simulink model "sat"  (R2019b)
settings: Solver=VariableStepAuto  StartTime=0.0  StopTime=T  RelTol=1e-3
values from neighbouring files (symbols this model uses):
  a0 = 2*Q + sinw    [filter_plot.m]    (also in sat_sim.m = (1 - cosw + sinw))
  a1 = -4*Q*cosw    [filter_plot.m]    (also in sat_sim.m = 2 * ( 1 - cosw))
  a2 = 2*Q - sinw    [filter_plot.m]    (also in sat_sim.m = 1 - cosw - sinw)
  b0 = Q*sinw    [filter_plot.m]    (also in sat_sim.m = 1 - cosw)
  b1 = 0    [filter_plot.m]    (also in sat_sim.m = 2 * b0)
  b2 = -Q*sinw    [filter_plot.m]    (also in sat_sim.m = b0)
  fs = 44100    [filter_plot.m]    (also in plot_adsr.m; plot_spectrogram.m; plot_waveform.m; sat_sim.m)
  G = 10.0    (= 10)    [sat_sim.m]
libraries: dspsrcs4 x3
settings Model: SimulationMode=rapid-accelerator  Creator=27849  LastModifiedBy=27849

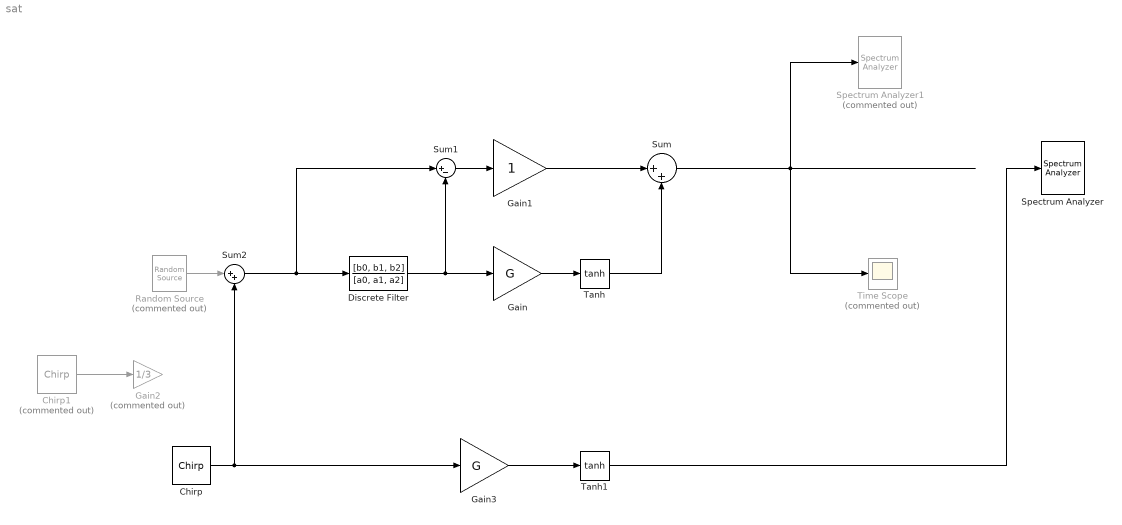
== system sat ==
  Chirp : dspsrcs4/Chirp  sweep=Logarithmic  mode=Unidirectional  f0=20  f1=20000  t1=T  Tsweep=T  phase=0  Ts=1/fs  spf=8096  datatype=Double  OutputFrames=off
      settings: SourceProductName=DSP System Toolbox
  Chirp1 : dspsrcs4/Chirp  Commented=on  sweep=Logarithmic  mode=Unidirectional  f0=60  f1=15000  t1=T  Tsweep=T  phase=0  Ts=1/fs  spf=8096  datatype=Double  OutputFrames=off
      settings: SourceProductName=DSP System Toolbox
  Discrete Filter : DiscreteFilter  Numerator=[b0, b1, b2]  Denominator=[a0, a1, a2]  InputProcessing=Columns as channels (frame based)
  Gain : Gain  Gain=G
  Gain1 : Gain
  Gain2 : Gain  Commented=on  Gain=1/3
  Gain3 : Gain  Gain=G
  Random Source : dspsrcs4/Random Source  Commented=on  SrcType=Uniform  NormMethod=Ziggurat  CltLength=12  MinVal=-1  MaxVal=1  MeanVal=0  VarVal=1  RepMode=Not repeatable  rawSeed=1  IsInherit=off  SampMode=Discrete  SampTime=1/fs  SampFrame=8096  DataType=Double  OutComplex=Real  OutputFrames=off
  Spectrum Analyzer : SpectrumAnalyzer
  Spectrum Analyzer1 : SpectrumAnalyzer  Commented=on
  Sum : Sum  Inputs=|++
  Sum1 : Sum  Inputs=|+-
  Sum2 : Sum  Inputs=|++
  Tanh : Trigonometry  Operator=tanh
  Tanh1 : Trigonometry  Operator=tanh
  Time Scope : Scope  Commented=on
  wires:
  Discrete Filter/1 -> Sum1/2, Gain/1
  Gain/1 -> Tanh/1
  Gain1/1 -> Sum/1
  Tanh/1 -> Sum/2
  Sum1/1 -> Gain1/1
  Sum/1 -> Time Scope/1, Spectrum Analyzer1/1
  Sum2/1 -> Sum1/1, Discrete Filter/1
  Chirp1/1 -> Gain2/1
  Random Source/1 -> Sum2/1
  Chirp/1 -> Gain3/1, Sum2/2
  Tanh1/1 -> Spectrum Analyzer/1
  Gain3/1 -> Tanh1/1
